simulink model "LandingSimulation"  (R2015a)
settings: Solver=ode45  StartTime=0.0  StopTime=10000  FixedStep=.5  RelTol=1e-5
values from neighbouring files (symbols this model uses):
  g0 = Planet_MU/Planet_Radius^2    (= 1.62845995)    [Constants.m]    (also in Constants_simple.m = 10)
  Planet_MU = 6.5138398E+10    (= 65138398000)    [Constants.m]
  Planet_Omega = 2*pi/138984.38    (= 4.52078521858e-05)    [Constants.m]
  Planet_Radius = 200000    [Constants.m]
  Starting_Alt = (Starting_Alt_High+Starting_Alt_Low)/2    (= 50000)    [Constants.m]    (also in SolverSuicideBurn_Base.m = (Starting_Alt_High+Starting_Alt_Low)/2)
  Starting_X_Speed = 100    [Constants_simple.m]    (also in StartingSpeed.m = V_per)
  Starting_Y_Speed = -25    [Constants_simple.m]    (also in StartingSpeed.m = 0)
  Terrain_Height = 0    [Constants.m]    (also in SolverSuicideBurn.m; SolverSuicideBurn_Terrain.m = Terrain_Height_plot(k))
  TWR = 2.5    [Constants_simple.m]    (also in SolverSuicideBurn.m = TWR_plot(j); SolverSuicideBurn_Terrain.m = TWR_plot(j))
libraries: simulink x2, vrlib x1
settings Model: Creator=raulm_000  LastModifiedBy=raulm_000

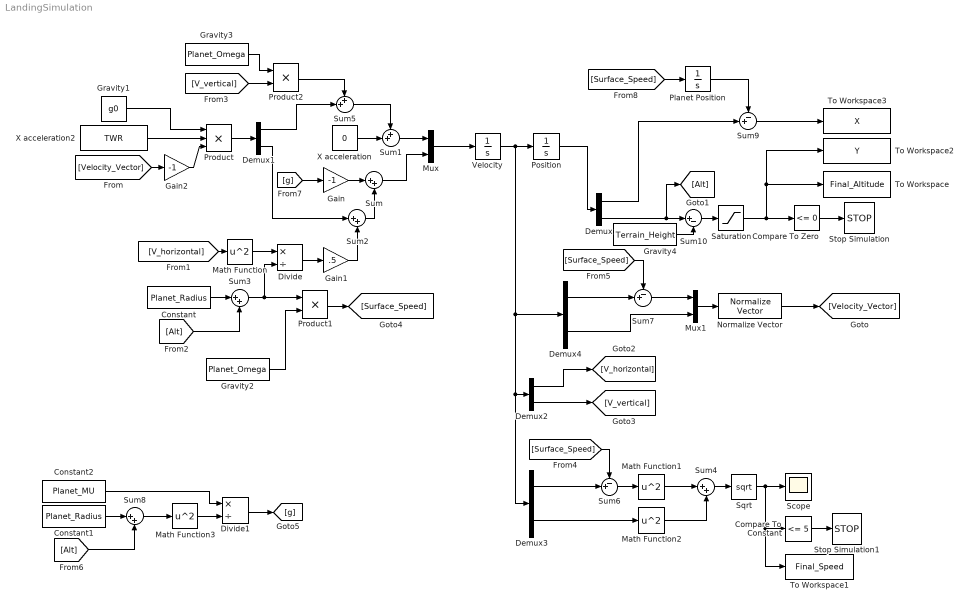
== system LandingSimulation ==
  Compare To Constant : simulink/Logic and Bit Operations/Compare To Constant  relop=<=  const=5  OutDataTypeStr=boolean
  Compare To Zero : simulink/Logic and Bit Operations/Compare To Zero  relop=<=  OutDataTypeStr=boolean
  Constant : Constant  Value=Planet_Radius
  Constant1 : Constant  Value=Planet_Radius
  Constant2 : Constant  Value=Planet_MU
  Demux{,1..4} (5 alike) : Demux  Outputs=2
  Divide : Product  Inputs=*/
  Divide1 : Product  Inputs=*/
  Gain : Gain  Gain=-1
  Gain1 : Gain  Gain=.5
  Gain2 : Gain  Gain=-1
  Gravity1 : Constant  Value=g0
  Gravity2 : Constant  Value=Planet_Omega
  Gravity3 : Constant  Value=Planet_Omega
  Gravity4 : Constant  Value=Terrain_Height
  Math Function{,1..3} (4 alike) : Math  Operator=square  SaturateOnIntegerOverflow=on
  Mux : Mux  Inputs=2
  Mux1 : Mux  Inputs=2
  Normalize Vector : vrlib/Utilities/Normalize Vector  maxzero=0
  Planet Position : Integrator
  Position : Integrator  InitialCondition=[0,Starting_Alt+Terrain_Height]
  Product : Product  Inputs=3
  Product1 : Product
  Product2 : Product
  Saturation : Saturate  UpperLimit=inf  LowerLimit=0
  Scope : Scope
      settings: YMin=9.96725e-07  YMax=9.96725e-07
  Sqrt : Sqrt  SaturateOnIntegerOverflow=on
  Stop Simulation : Stop
  Stop Simulation1 : Stop
  Sum{,2..4,8} (5 alike) : Sum  Inputs=|++
  Sum1 : Sum  Inputs=++|
  Sum10 : Sum  Inputs=|+-
  Sum5 : Sum  Inputs=++|
  Sum6 : Sum  Inputs=-+|
  Sum7 : Sum  Inputs=-+|
  Sum9 : Sum  Inputs=-+|
  To Workspace : ToWorkspace  VariableName=Final_Altitude  SampleTime=-1
      settings: MaxDataPoints=1
  To Workspace1 : ToWorkspace  VariableName=Final_Speed  SampleTime=-1
      settings: MaxDataPoints=1
  To Workspace2 : ToWorkspace  VariableName=Y  SampleTime=-1
  To Workspace3 : ToWorkspace  VariableName=X  SampleTime=-1
  Velocity : Integrator  InitialCondition=[Starting_X_Speed,Starting_Y_Speed]
  X acceleration : Constant  Value=0
  X acceleration2 : Constant  Value=TWR
  wires:
  Mux/1 -> Velocity/1
  [g] -> Gain/1
  Position/1 -> Demux/1
  Compare To Zero/1 -> Stop Simulation/1
  Normalize Vector/1 -> [Velocity_Vector]
  Gain/1 -> Sum/1
  Sum/1 -> Mux/2
  X acceleration/1 -> Sum1/2
  Sum1/1 -> Mux/1
  Velocity/1 -> Demux4/1, Demux2/1, Demux3/1, Position/1
  Demux2/1 -> [V_horizontal]
  Product/1 -> Demux1/1
  Demux1/2 -> Sum2/1
  Sum2/1 -> Sum/2
  [V_horizontal] -> Math Function/1
  Constant/1 -> Sum3/1
  [Alt] -> Sum3/2
  Math Function/1 -> Divide/1
  Sum3/1 -> Product1/1, Divide/2
  Divide/1 -> Gain1/1
  Demux2/2 -> [V_vertical]
  Demux3/2 -> Math Function2/1
  Math Function1/1 -> Sum4/1
  Math Function2/1 -> Sum4/2
  Sum4/1 -> Sqrt/1
  Sqrt/1 -> Compare To Constant/1, To Workspace1/1, Scope/1
  Compare To Constant/1 -> Stop Simulation1/1
  Gain1/1 -> Sum2/2
  [Velocity_Vector] -> Gain2/1
  X acceleration2/1 -> Product/2
  Gain2/1 -> Product/3
  Gravity1/1 -> Product/1
  Sum5/1 -> Sum1/1
  Demux1/1 -> Sum5/2
  [V_vertical] -> Product2/2
  Product2/1 -> Sum5/1
  Gravity2/1 -> Product1/2
  Product1/1 -> [Surface_Speed]
  Sum6/1 -> Math Function1/1
  Demux3/1 -> Sum6/2
  [Surface_Speed] -> Sum6/1
  Gravity3/1 -> Product2/1
  Demux4/1 -> Sum7/2
  [Surface_Speed] -> Sum7/1
  Demux4/2 -> Mux1/2
  Sum7/1 -> Mux1/1
  Mux1/1 -> Normalize Vector/1
  Math Function3/1 -> Divide1/2
  Constant1/1 -> Sum8/1
  [Alt] -> Sum8/2
  Sum8/1 -> Math Function3/1
  Constant2/1 -> Divide1/1
  Divide1/1 -> [g]
  [Surface_Speed] -> Planet Position/1
  Demux/1 -> Sum9/2
  Sum9/1 -> To Workspace3/1
  Planet Position/1 -> Sum9/1
  Demux/2 -> Sum10/1, [Alt]
  Gravity4/1 -> Sum10/2
  Sum10/1 -> Saturation/1
  Saturation/1 -> To Workspace/1, To Workspace2/1, Compare To Zero/1
